simulink model "main"  (R2023a)
settings: Solver=ode23  StartTime=0.0  StopTime=8  RelTol=1e-3
settings Model: Creator=ycheb  LastModifiedBy=ycheb

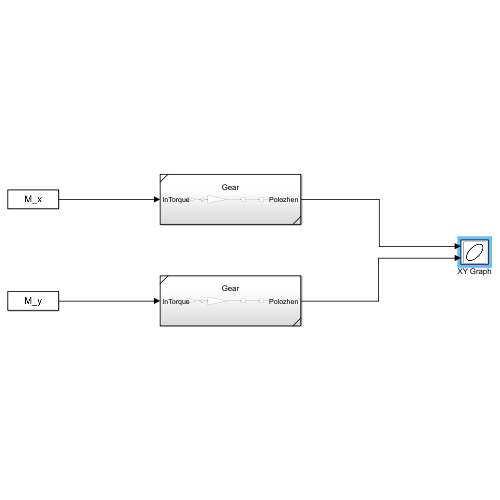
[thumbnail: Simulink's stored preview of the top-level diagram]
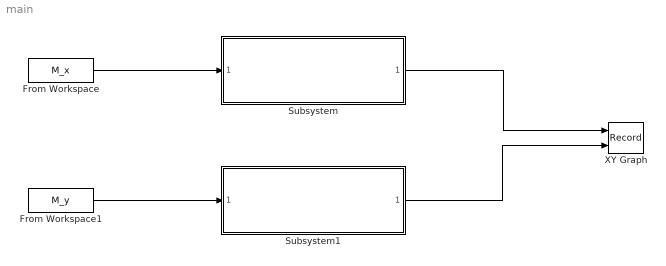
== system main ==
  From Workspace : FromWorkspace  VariableName=M_x  OutputAfterFinalValue=Setting to zero
  From Workspace1 : FromWorkspace  VariableName=M_y  OutputAfterFinalValue=Setting to zero
  Subsystem : Subsystem  ReferencedSubsystem=Gear
  Subsystem1 : Subsystem  ReferencedSubsystem=Gear
  XY Graph : Record  FileSettingsInternal="{\"entries\":[{\"content\":{\"excelSettings\":{\"content\":{},\"type\":\"Streamout.ExcelSettings\"}},\"type\":\"Streamout.FileSettingStorage\",\"uuid\":\"\"}],\"packageUris\":[\"http:\\/\\/schema.mathworks.com\\/mf0\\/streamout_blocks\\/R2020a\"],\"version\":\"1.0\"}"  Layout=[1 1]  SignalsInternal="{\"entries\":[{\"content\":{\"signals\":[{\"content\":{\"blockPath\":[],\"dimensions\":[1],\"domain\":\"\",\"lineColor\":\"#a2142f\",\"plots\":[1],\"port\":1,\"sid\":[\"\"],\"signalID\":258,\"signalName\":\"Subsystem\"},\"type\":\"RecordBlkView.Signal\",\"uuid\":\"\"},{\"content\":{\"blockPath\":[],\"dimensions\":[1],\"domain\":\"\",\"lineColor\":\"#139fff\",\"plots\":[1],\"port\":2,\"sid\":[\"\"],\"signalID\":262,\"signalName\":\"Subsystem1\"},\"type\":\"RecordBlkView.Signal\",\"uuid\":\"\"}]},\"type\":\"RecordBlkView.InputSignals\",\"uuid\":\"\"}],\"packageUris\":[\"http:\\/\\/schema.mathworks.com\\/mf0\\/streamout_blocks\\/R2020a\"],\"version\":\"1.0\"}"  VisualizationBindings="{\"xyplotplugin\":{\"info\":[{\"series\":[{\"bindingParametersList\":[{\"parameter\":\"X-Axis\",\"signalID\":258,\"signalName\":\"Subsystem\"},{\"parameter\":\"Y-Axis\",\"signalID\":262,\"signalName\":\"Subsystem1\"}],\"seriesID\":54452}],\"subplotID\":1}]}}"  CompatibilityTag=XY
  wires:
  Subsystem1/1 -> XY Graph/2
  From Workspace/1 -> Subsystem/1
  Subsystem/1 -> XY Graph/1
  From Workspace1/1 -> Subsystem1/1
